simulink model "natural_frequency_comparison"  (R2021b)
settings: Solver=VariableStepAuto  StartTime=0.0  StopTime=30  RelTol=1e-3
settings Model: Creator=admin  LastModifiedBy=admin

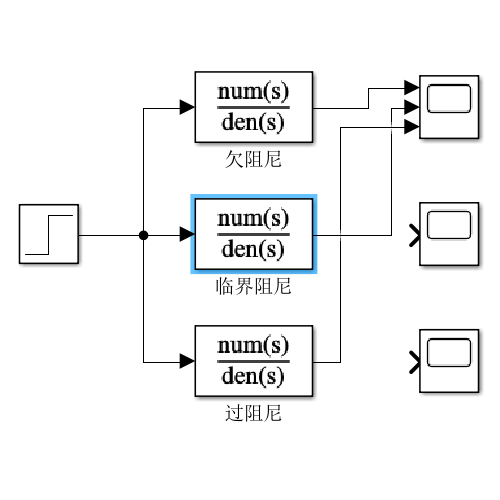
[thumbnail: Simulink's stored preview of the top-level diagram]
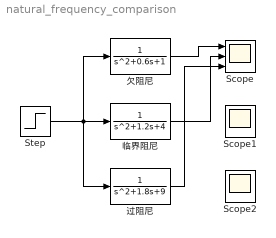
== system natural_frequency_comparison ==
  Scope : Scope  NumInputPorts=3
  Scope1 : Scope
  Scope2 : Scope
  Step : Step  SampleTime=0
  临界阻尼 : TransferFcn  Denominator=[1,1.2, 4]
  欠阻尼 : TransferFcn  Denominator=[1,0.6,1]
  过阻尼 : TransferFcn  Denominator=[1,1.8,9]
  wires:
  欠阻尼/1 -> Scope/1
  Step/1 -> 欠阻尼/1, 过阻尼/1, 临界阻尼/1
  临界阻尼/1 -> Scope/2
  过阻尼/1 -> Scope/3
